simulink model "torbk2_m"  (Simulink 7.9)
settings: Solver=ode45  SolverMode=SingleTasking  StartTime=0.0  StopTime=999999  MaxStep=10  RelTol=1e-3  AbsTol=1e-3
values from neighbouring files (symbols this model uses):
  U = st_Varia('ShortNames')    [torbk2_i.m]    (also in torbsc_i.m)
  x0 = [0.00001;zeros(NumCel-1,1);zeros(NumCel,1);0.0000005*ones(NumCel,1);zeros(NumCel,1);zeros(NumCel,1);0;0;0;0;0;zeros(NumCel,1);0.0002*ones(NumCel,1);zeros(NumCel,1);zeros(NumCel,1);zeros(NumCel,1);zeros(NumCel,1)]    [torbk2_i.m]    (also in torbk2_s.m = x0; torbsc_i.m; torbsc_s.m = x0)
undefined symbols (not defined in the file or in its folder): B
settings Model: Creator=M.Sparnaaij  LastModifiedBy=M.Sparnaaij
settings DataIOCC: LimitDataPoints=off  SaveOutput=off  SaveTime=off  SignalLoggingName=sigsOut
settings OptimizationCC: BooleanDataType=off
settings DebuggingCC: SaveWithParameterizedLinksMsg=none  SignalResolutionControl=TryResolveAllWithWarning  SolverPrmCheckMsg=none  MultiTaskDSMMsg=warning  MultiTaskCondExecSysMsg=none  StrictBusMsg=None
settings HardwareCC: TargetUnknown=on
settings RTWCC: IncludeERTFirstTime=on
settings GRTTargetCC: CombineOutputUpdateFcns=off  GRTInterface=on

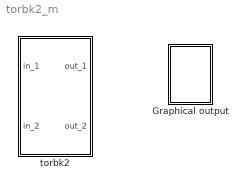
== system torbk2_m ==
  Graphical output : Subsystem
      settings: OpenFcn=torbk2_g
      mask Display:
      | plot(0,0,100,100,[80,20,20],[20,20,80],[80,69,60,52,45,39,33,28,24,20],[65,65,64,61,57,52,45,37,30,20])
      | disp('');
      | text(100,100,'torbk2', 'horizontalAlignment', 'right', 'verticalAlignment', 'top');
  torbk2 : Subsystem  Description=This model calculates the aeration and degassifying with a packed column aerator. The influent carbon dioxide concentration is calculated on the basis of the bicarbonate concentration, the pH, the EGV and the water temperature, so these parameters must always be filled out in the 'Water quality parameters' block.
      mask init:
      | filenaam='.\StimelaData\Packed_column_aerator_sc.mat';
      | 
      | [Pn,Fn,Fext]=Fileprop(filenaam);
      | 
      | errstr = st_UniqName(filenaam,'filenaam=''','SubSystem','OpenFcn');
      | if errstr, error([errstr 'The filename "' filenaam '" is already in use. Choose a different filename.']), end
      | 
      | P = torbk2_p(filenaam);
      | [B,x0,U]=torbk2_i(filenaam);
      settings: OpenFcn=|
      | filenaam='.\StimelaData\Packed_column_aerator_sc.mat';
      | st_ParameterInput('init',gcb,filenaam,'torbk2');
      mask Display:
      | plot(0,0,100,100,[20,20],[20,80],[80,80],[20,80],[20,80,20,80,20],[30,70,70,30,30],[80,20],[28,28],[50,44,34,27,23,20],[90,90,89,87,84,80],[50,44,34,27,23,20],[10,10,11,13,16,20],[50,56,66,73,77,80],[90,90,89,87,84,80],[50,56,66,73,77,80],[10,10,11,13,16,20],[21,20],[82,80],[10,50,50,10],[82,82,80,80],[58,50,42],[76,80,76],[50,35,45,45],[99,94,94,90],[50,65,55,55],[99,94,94,90],[45,45],[3,10],[55,55],[3,10])
      | disp('')
      | text(50,50,'torbk2', 'horizontalAlignment', 'center', 'verticalAlignment', 'middle');
      | text(50,0,Fn, 'horizontalAlignment', 'center', 'verticalAlignment', 'base');

== system torbk2_m/Graphical output ==
  note: plotten

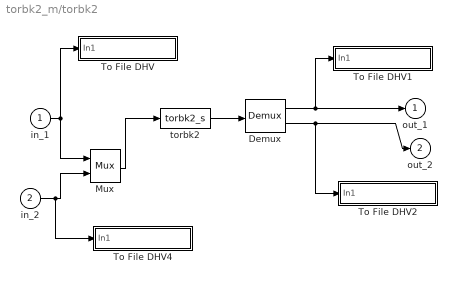
== system torbk2_m/torbk2 ==
  in_1 : Inport
  in_2 : Inport  Port=2
  Demux : Demux  Outputs=[U.Number B.Measurements]
  Mux : Mux  Inputs=[U.Number B.Setpoints]
  To File DHV : Subsystem  mask(To File DHV){naam=[filenaam(1:length(filenaam)-4) '_in.sti']}
      mask prompts: naam "Naam van bestand"
      mask init:
      | set_param([gcb '/To File'],'Filename',naam);
      mask Display: disp(naam)
  To File DHV1 : Subsystem  mask(To File DHV){naam=[filenaam(1:length(filenaam)-4) '_out.sti']}
      mask prompts: naam "Naam van bestand"
      mask init:
      | set_param([gcb '/To File'],'Filename',naam);
      mask Display: disp(naam)
  To File DHV2 : Subsystem  mask(To File DHV){naam=[filenaam(1:length(filenaam)-4) '_EM.sti']}
      mask prompts: naam "Naam van bestand"
      mask init:
      | set_param([gcb '/To File'],'Filename',naam);
      mask Display: disp(naam)
  To File DHV4 : Subsystem  mask(To File DHV){naam=[filenaam(1:length(filenaam)-4) '_ES.sti']}
      mask prompts: naam "Naam van bestand"
      mask init:
      | set_param([gcb '/To File'],'Filename',naam);
      mask Display: disp(naam)
  torbk2 : S-Function  FunctionName=torbk2_s  Parameters=B,x0,U,P  EnableBusSupport=off
  out_1 : Outport  InitialOutput=0
  out_2 : Outport  Port=2  InitialOutput=0
  wires:
  in_1/1 -> To File DHV/1(In1), Mux/1
  Demux/2 -> To File DHV2/1(In1), out_2/1
  Demux/1 -> To File DHV1/1(In1), out_1/1
  torbk2/1 -> Demux/1
  in_2/1 -> Mux/2, To File DHV4/1(In1)
  Mux/1 -> torbk2/1

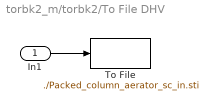
== system torbk2_m/torbk2/To File DHV ==
  In1 : Inport
  To File : ToFile  Filename=./Packed_column_aerator_sc_in.sti  MatrixName=torbk2in
  wires:
  In1/1 -> To File/1

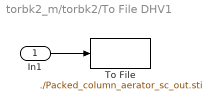
== system torbk2_m/torbk2/To File DHV1 ==
  In1 : Inport
  To File : ToFile  Filename=./Packed_column_aerator_sc_out.sti  MatrixName=torbk2out
  wires:
  In1/1 -> To File/1

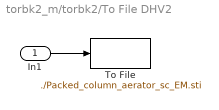
== system torbk2_m/torbk2/To File DHV2 ==
  In1 : Inport
  To File : ToFile  Filename=./Packed_column_aerator_sc_EM.sti  MatrixName=torbk2EM
  wires:
  In1/1 -> To File/1

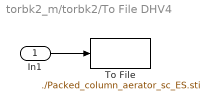
== system torbk2_m/torbk2/To File DHV4 ==
  In1 : Inport
  To File : ToFile  Filename=./Packed_column_aerator_sc_ES.sti  MatrixName=torbk2ES
  wires:
  In1/1 -> To File/1
